simulink model "sl_mobile_vs_omni"  (R2015b)
settings: Solver=ode45  StartTime=0.0  StopTime=10  RelTol=1e-3
InitFcn:
  | camera = CentralCamera('default', 'name', 'mobile_vs', 'focal', 0.002);
  | T_vc = transl(0.2, 0.1, 0.3)*troty(pi/2)*trotz(-pi/2); %*trotx(-pi/4);
  | P = [0 0; 1 -1; 2 2];
  | pstar = camera.project(P, 'Tcam', transl(-2, 0, 0)*T_vc);
libraries: roblocks x8, simulink x1
settings Model: ExtModeTrigMode=oneshot  ExtModeArmWhenConnect=off  Creator=pic  LastModifiedBy=corkep
settings DataIOCC: LimitDataPoints=off  SaveFormat=Structure  SignalLoggingSaveFormat=ModelDataLogs  ReturnWorkspaceOutputs=on
settings OptimizationCC: BlockReduction=off  BooleanDataType=off  ExpressionDepthLimit=2147483647  InitFltsAndDblsToZero=on
settings DebuggingCC: SaveWithParameterizedLinksMsg=none  UnderspecifiedInitializationDetection=Classic  MergeDetectMultiDrivingBlocksExec=none  SignalResolutionControl=TryResolveAllWithWarning  MultiTaskDSMMsg=warning  MultiTaskCondExecSysMsg=none  FcnCallInpInsideContextMsg=UseLocalSettings  StateNameClashWarn=warning
settings HardwareCC: ProdBitPerPointer=32  ProdLargestAtomicFloat=None  ProdIntDivRoundTo=Undefined  ProdEndianess=Unspecified  ProdWordSize=32  ProdHWDeviceType=32-bit Generic  TargetUnknown=on
settings GRTTargetCC: ModelReferenceCompliant=off  CompOptLevelCompliant=off  GeneratePreprocessorConditionals=Disable all  CombineOutputUpdateFcns=off  MatFileLogging=off  GRTInterface=on
settings ConfigComp: CovModelRefEnable=Off  CovSFcnEnable=off

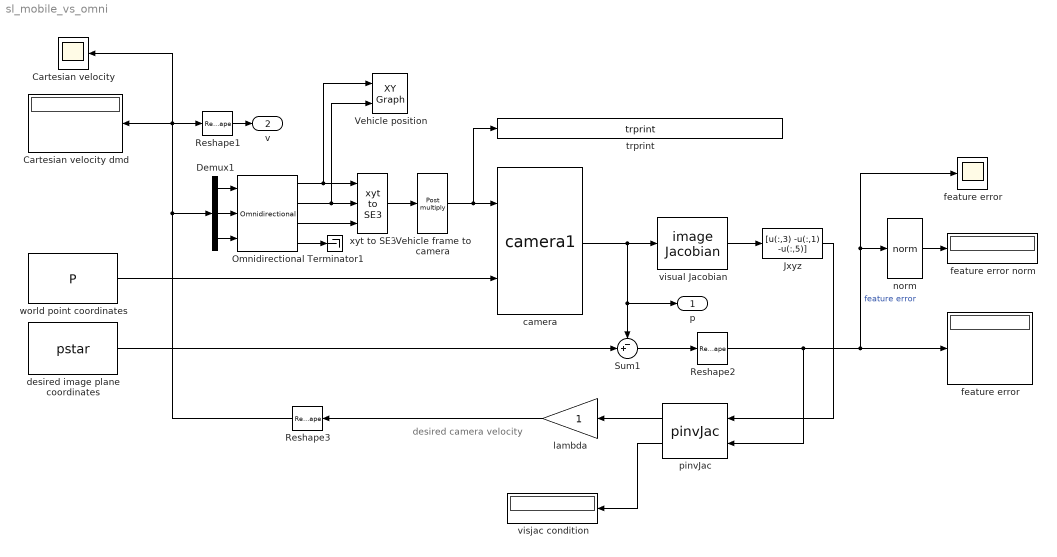
== system sl_mobile_vs_omni ==
  note: desired camera velocity
  Cartesian velocity : Scope
  Cartesian velocity dmd : Display
      settings: Format=bank
  Demux1 : Demux  Outputs=3
  Jxyz : MATLABFcn  MATLABFcn=[u(:,3) -u(:,1) -u(:,5)]  Output1D=off
  Omnidirectional : roblocks/Vehicles/Omnidirectional  accel=1  vlim=1  alim=2  L=0  x0=[-8 2 0.3]  P=[1 1 -1 -1; 1 -1 -1 1]  alpha=[1 -1 1 -1]*pi/4  R=0.1
  Reshape1 : Reshape  OutputDimensions=6
  Reshape2 : Reshape  OutputDimensions=6
  Reshape3 : Reshape  OutputDimensions=6
  Sum1 : Sum  Inputs=-+|  SaturateOnIntegerOverflow=on  InputSameDT=on  OutDataTypeStr=Inherit: Same as first input
  Terminator1 : Terminator
  Vehicle frame to camera : roblocks/Toolbox/Post multiply  T2=T_vc
  Vehicle position : simulink/Sinks/XY Graph  xmin=-10  xmax=10  ymin=-10  ymax=10  st=-1
  camera : roblocks/Vision/camera1  cam=camera
  desired image plane coordinates : Constant  Value=pstar  VectorParams1D=off
  feature error : Display
      settings: Format=bank
  feature error norm : Display
  "feature error " : Scope
  lambda : Gain  SaturateOnIntegerOverflow=on  OutDataTypeStr=Inherit: Same as input  ParamDataTypeStr=Inherit: Same as input
  norm : roblocks/Toolbox/norm  SystemSampleTime=-1
  pinvJac : roblocks/Toolbox/pinvJac
  trprint : roblocks/Toolbox/trprint  options={}
      link override S-Function: Parameters=options
  visjac condition : Display
  visual Jacobian : roblocks/Vision/image Jacobian  cam=camera  z=3
  world point coordinates : Constant  Value=P  VectorParams1D=off
  xyt to SE3 : roblocks/Toolbox/xyt to SE3
  p : Outport
  v : Outport  Port=2
  wires:
  Sum1/1 -> Reshape2/1
  desired image plane coordinates/1 -> Sum1/2
  Reshape2/1 -> "feature error "/1, norm/1, feature error/1, pinvJac/2  "feature error"
  pinvJac/2 -> visjac condition/1
  pinvJac/1 -> lambda/1
  visual Jacobian/1 -> Jxyz/1
  lambda/1 -> Reshape3/1
  Reshape1/1 -> v/1
  camera/1 -> visual Jacobian/1, Sum1/1, p/1
  world point coordinates/1 -> camera/2
  norm/1 -> feature error norm/1
  Jxyz/1 -> pinvJac/1
  Vehicle frame to camera/1 -> trprint/1, camera/1
  Reshape3/1 -> Reshape1/1, Cartesian velocity/1, Cartesian velocity dmd/1, Demux1/1
  Demux1/1 -> Omnidirectional/1
  Demux1/2 -> Omnidirectional/2
  Demux1/3 -> Omnidirectional/3
  Omnidirectional/1 -> xyt to SE3/1, Vehicle position/1
  Omnidirectional/2 -> xyt to SE3/2, Vehicle position/2
  xyt to SE3/1 -> Vehicle frame to camera/1
  Omnidirectional/4 -> Terminator1/1
  Omnidirectional/3 -> xyt to SE3/3
